simulink model "b1"  (R2020b)
settings: Solver=VariableStepAuto  StartTime=0.0  StopTime=50.0  RelTol=1e-3
settings Model: Creator=Marco  LastModifiedBy=Marco

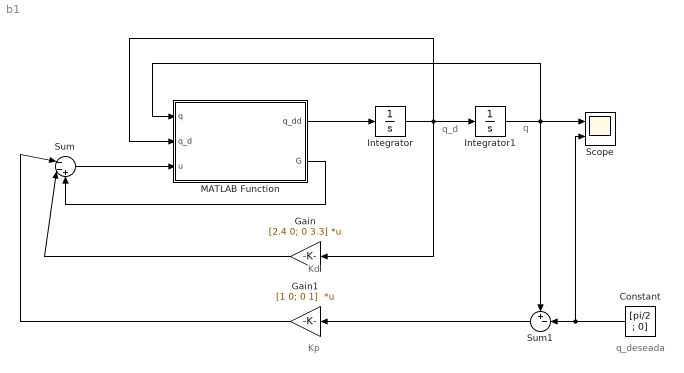
== system b1 ==
  note: q_deseada
  note: q
  note: q_d
  note: Kd
  note: Kp
  Constant : Constant  Value=[pi/2 ; 0]
  Gain : Gain  Gain=[2.4 0; 0 3.3]  Multiplication=Matrix(K*u)
  Gain1 : Gain  Gain=[1 0; 0 1]  Multiplication=Matrix(K*u)
  Integrator : Integrator  InitialCondition=[0; 0]
  Integrator1 : Integrator  InitialCondition=[0; 0]
  MATLAB Function : MATLAB Function  TreatAsAtomicUnit=on
  Scope : Scope  NumInputPorts=2
  Sum : Sum  Inputs=|--+
  Sum1 : Sum  Inputs=+-|
  wires:
  MATLAB Function/1(q_dd) -> Integrator/1
  Integrator/1 -> MATLAB Function/2(q_d), Gain/1, Integrator1/1
  Sum/1 -> MATLAB Function/3(u)
  MATLAB Function/2(G) -> Sum/3
  Gain/1 -> Sum/2
  Gain1/1 -> Sum/1
  Sum1/1 -> Gain1/1
  Integrator1/1 -> MATLAB Function/1(q), Scope/1, Sum1/1
  Constant/1 -> Scope/2, Sum1/2

== matlab function b1/MATLAB Function ==
  data: q input; q_d input; u input; q_dd output; G output
function [q_dd, G] = manipulador(q, q_d, u)

I1 = 0.5; m1 = 0.5; L1 = 0.5; Lc1 = 0.25; 
I2 = 0.3; m2 = 0.3; L2 = 0.3; Lc2 = 0.15; g = 9.8;

M11 = m1*Lc1^2 + I1 + m2*[L1^2 + Lc2^2 + 2*L1*Lc2*cos(q(2))] + I2;
M22 = m2*Lc2^2 + I2;
M12 = m2*L1*Lc2*cos(q(2)) + m2*Lc2^2 + I2;
C11 = -(m2*L1*Lc2*sin(q(2)))*q_d(2);
C12 = -(m2*L1*Lc2*sin(q(2)))*q_d(1) + C11;
C21 = (m2*L1*Lc2*sin(q(2)))*q_d(1);
g1 = m1*Lc1*g*cos(q(1)) + m2*g*(Lc2*cos(q(1) + q(2)) + L1*cos(q(1)));
g2 = m2*g*Lc2*cos(q(1) + q(2));

M = [M11 M12;
     M12 M22];
C = [C11 C12;
     C21  0 ];
G = [g1; g2];

q_dd = M\(u-C*q_d-G);

end
